simulink library "bus_stubs_fsw"  (R2016b)
settings: Solver=VariableStepAuto  StartTime=0.0  StopTime=10.0  RelTol=1e-3
settings Model: Creator=taylorreynolds  LastModifiedBy=taylorreynolds

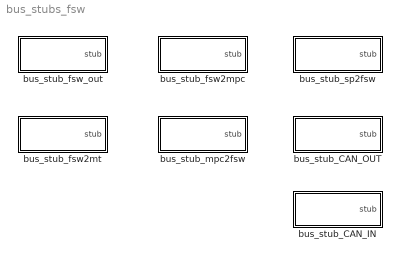
== system bus_stubs_fsw ==
  bus_stub_CAN_IN : Subsystem
      mask help: Creates bus compliant with actuatorCmd (actuator command) bus object.
      mask Help: Provides a zeroed bus which complies with the actuatorCmd bus object.
      mask DialogControl DescGroupVar Prompt: bus_stub_actCmd
      mask DialogControl DescTextVar Prompt: Creates bus compliant with actuatorCmd (actuator command) bus object.
  bus_stub_CAN_OUT : Subsystem
      mask help: Creates bus compliant with actuatorCmd (actuator command) bus object.
      mask Help: Provides a zeroed bus which complies with the actuatorCmd bus object.
      mask DialogControl DescGroupVar Prompt: bus_stub_actCmd
      mask DialogControl DescTextVar Prompt: Creates bus compliant with actuatorCmd (actuator command) bus object.
  bus_stub_fsw2mpc : Subsystem
      mask help: Creates bus compliant with actuatorCmd (actuator command) bus object.
      mask Help: Provides a zeroed bus which complies with the actuatorCmd bus object.
      mask DialogControl DescGroupVar Prompt: bus_stub_actCmd
      mask DialogControl DescTextVar Prompt: Creates bus compliant with actuatorCmd (actuator command) bus object.
  bus_stub_fsw2mt : Subsystem
      mask help: Creates bus compliant with actuatorCmd (actuator command) bus object.
      mask Help: Provides a zeroed bus which complies with the actuatorCmd bus object.
      mask DialogControl DescGroupVar Prompt: bus_stub_actCmd
      mask DialogControl DescTextVar Prompt: Creates bus compliant with actuatorCmd (actuator command) bus object.
  bus_stub_fsw_out : Subsystem
      mask help: Creates bus compliant with actuatorCmd (actuator command) bus object.
      mask Help: Provides a zeroed bus which complies with the actuatorCmd bus object.
      mask DialogControl DescGroupVar Prompt: bus_stub_actCmd
      mask DialogControl DescTextVar Prompt: Creates bus compliant with actuatorCmd (actuator command) bus object.
  bus_stub_mpc2fsw : Subsystem
      mask help: Creates bus compliant with actuatorCmd (actuator command) bus object.
      mask Help: Provides a zeroed bus which complies with the actuatorCmd bus object.
      mask DialogControl DescGroupVar Prompt: bus_stub_actCmd
      mask DialogControl DescTextVar Prompt: Creates bus compliant with actuatorCmd (actuator command) bus object.
  bus_stub_sp2fsw : Subsystem
      mask help: Creates bus compliant with actuatorCmd (actuator command) bus object.
      mask Help: Provides a zeroed bus which complies with the actuatorCmd bus object.
      mask DialogControl DescGroupVar Prompt: bus_stub_actCmd
      mask DialogControl DescTextVar Prompt: Creates bus compliant with actuatorCmd (actuator command) bus object.

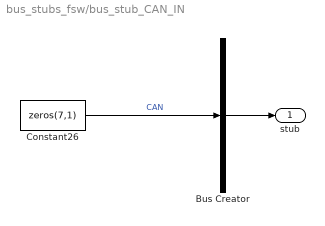
== system bus_stubs_fsw/bus_stub_CAN_IN ==
  Bus Creator : BusCreator  Inputs=1
  Constant26 : Constant  Value=zeros(7,1)
  stub : Outport  OutDataTypeStr=Bus: CAN_IN
  wires:
  Constant26/1 -> Bus Creator/1  "CAN"
  Bus Creator/1 -> stub/1

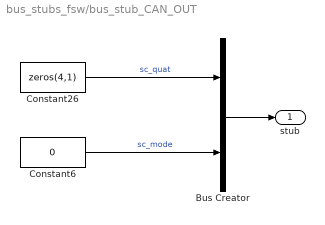
== system bus_stubs_fsw/bus_stub_CAN_OUT ==
  Bus Creator : BusCreator  Inputs=2
  Constant26 : Constant  Value=zeros(4,1)
  Constant6 : Constant  Value=0
  stub : Outport  OutDataTypeStr=Bus: CAN_OUT
  wires:
  Bus Creator/1 -> stub/1
  Constant6/1 -> Bus Creator/2  "sc_mode"
  Constant26/1 -> Bus Creator/1  "sc_quat"

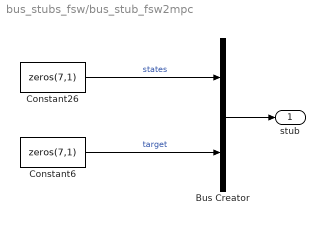
== system bus_stubs_fsw/bus_stub_fsw2mpc ==
  Bus Creator : BusCreator  Inputs=2
  Constant26 : Constant  Value=zeros(7,1)
  Constant6 : Constant  Value=zeros(7,1)
  stub : Outport  OutDataTypeStr=Bus: fsw2mpc
  wires:
  Bus Creator/1 -> stub/1
  Constant6/1 -> Bus Creator/2  "target"
  Constant26/1 -> Bus Creator/1  "states"

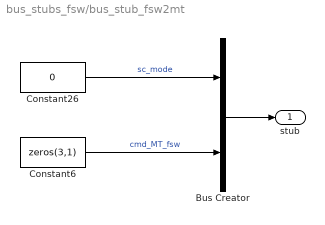
== system bus_stubs_fsw/bus_stub_fsw2mt ==
  Bus Creator : BusCreator  Inputs=2
  Constant26 : Constant  Value=0
  Constant6 : Constant  Value=zeros(3,1)
  stub : Outport  OutDataTypeStr=Bus: fsw2mt
  wires:
  Constant26/1 -> Bus Creator/1  "sc_mode"
  Constant6/1 -> Bus Creator/2  "cmd_MT_fsw"
  Bus Creator/1 -> stub/1

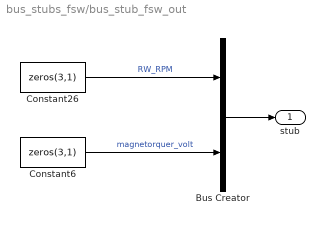
== system bus_stubs_fsw/bus_stub_fsw_out ==
  Bus Creator : BusCreator  Inputs=2
  Constant26 : Constant  Value=zeros(3,1)
  Constant6 : Constant  Value=zeros(3,1)
  stub : Outport  OutDataTypeStr=Bus: fsw_out
  wires:
  Constant26/1 -> Bus Creator/1  "RW_RPM"
  Constant6/1 -> Bus Creator/2  "magnetorquer_volt"
  Bus Creator/1 -> stub/1

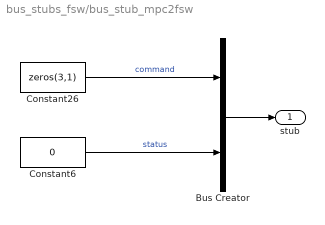
== system bus_stubs_fsw/bus_stub_mpc2fsw ==
  Bus Creator : BusCreator  Inputs=2
  Constant26 : Constant  Value=zeros(3,1)
  Constant6 : Constant  Value=0
  stub : Outport  OutDataTypeStr=Bus: mpc2fsw
  wires:
  Constant26/1 -> Bus Creator/1  "command"
  Constant6/1 -> Bus Creator/2  "status"
  Bus Creator/1 -> stub/1

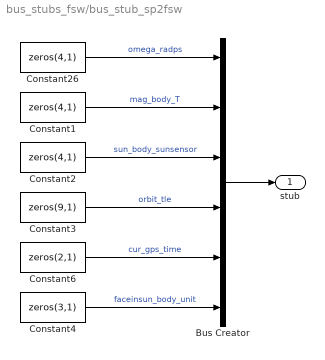
== system bus_stubs_fsw/bus_stub_sp2fsw ==
  Bus Creator : BusCreator  Inputs=6
  Constant1 : Constant  Value=zeros(4,1)
  Constant2 : Constant  Value=zeros(4,1)
  Constant26 : Constant  Value=zeros(4,1)
  Constant3 : Constant  Value=zeros(9,1)
  Constant4 : Constant  Value=zeros(3,1)
  Constant6 : Constant  Value=zeros(2,1)
  stub : Outport  OutDataTypeStr=Bus: sp2fsw
  wires:
  Bus Creator/1 -> stub/1
  Constant26/1 -> Bus Creator/1  "omega_radps"
  Constant1/1 -> Bus Creator/2  "mag_body_T"
  Constant2/1 -> Bus Creator/3  "sun_body_sunsensor"
  Constant3/1 -> Bus Creator/4  "orbit_tle"
  Constant6/1 -> Bus Creator/5  "cur_gps_time"
  Constant4/1 -> Bus Creator/6  "faceinsun_body_unit"
